simulink library "createRegressorMatrix"  (R2018a)
settings: Solver=VariableStepAuto  StartTime=0.0  StopTime=10.0  RelTol=1e-3
undefined symbols (not defined in the file): ctrl
libraries: createQuatraticRegressorVector x1, normalizeBasisParameters x1
settings Model: Creator=mitch  LastModifiedBy=mitch

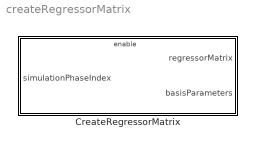
== system createRegressorMatrix ==
  CreateRegressorMatrix : Subsystem

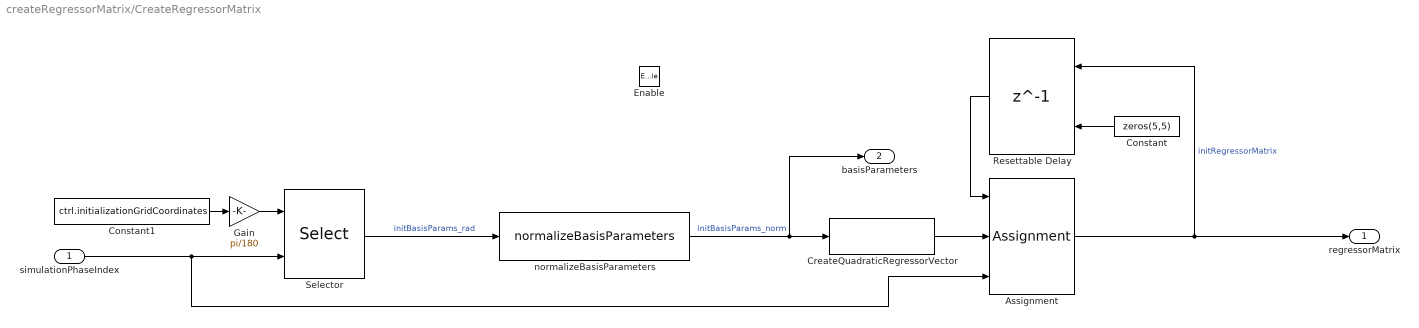
== system createRegressorMatrix/CreateRegressorMatrix ==
  simulationPhaseIndex : Inport
  Enable : EnablePort
  Assignment : Assignment  NumberOfDimensions=2  DiagnosticForDimensions=Warning  IndexOptions=Index vector (port),Assign all  Indices=1,1:5  OutputSizes=5,5
  Constant : Constant  Value=zeros(5,5)
  Constant1 : Constant  Value=ctrl.initializationGridCoordinates
  CreateQuadraticRegressorVector : createQuatraticRegressorVector/CreateQuadraticRegressorVector
  Gain : Gain  Gain=pi/180
  Resettable Delay : Delay  DelayLength=1  InitialConditionSource=Input port
      settings: InputPortMap=u0,p4
  Selector : Selector  NumberOfDimensions=2  InputPortWidth=3  IndexOptions=Index vector (port),Select all  Indices=[1 3],1:2  OutputSizes=1,1
  normalizeBasisParameters : normalizeBasisParameters/normalizeBasisParameters
  regressorMatrix : Outport
  basisParameters : Outport  Port=2  InitialOutput=([ctrl.width ctrl.height])./([ctrl.azimuthNormalizationFactor_deg ctrl.zenithNormalizationFactor_deg])
  wires:
  Selector/1 -> normalizeBasisParameters/1  "initBasisParams_rad"
  normalizeBasisParameters/1 -> CreateQuadraticRegressorVector/1, basisParameters/1  "initBasisParams_norm"
  simulationPhaseIndex/1 -> Assignment/3, Selector/2
  Resettable Delay/1 -> Assignment/1
  Constant/1 -> Resettable Delay/2
  Assignment/1 -> Resettable Delay/1, regressorMatrix/1  "initRegressorMatrix"
  CreateQuadraticRegressorVector/1 -> Assignment/2
  Gain/1 -> Selector/1
  Constant1/1 -> Gain/1
